simulink model "part_2_no_coulomb_friction"  (R2019a)
settings: Solver=VariableStepAuto  StartTime=0.0  StopTime=9  RelTol=1e-3
settings Model: Creator=Matthew Frantz  LastModifiedBy=Matthew Frantz
settings SolverCC: ZeroCrossAlgorithm=Adaptive
settings DebuggingCC: IgnoredZcDiagnostic=none

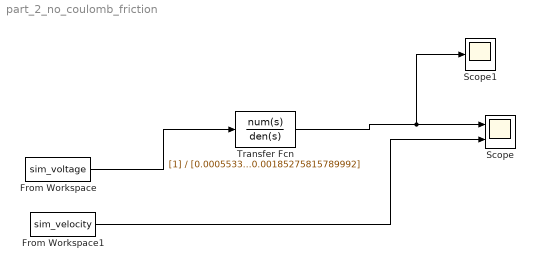
== system part_2_no_coulomb_friction ==
  From Workspace : FromWorkspace  VariableName=sim_voltage  OutDataTypeStr=double  SampleTime=0.001
  From Workspace1 : FromWorkspace  VariableName=sim_velocity  SampleTime=0.001
  Scope : Scope  NumInputPorts=2
  Scope1 : Scope
  Transfer Fcn : TransferFcn  Denominator=[0.000553342193254858 0.00185275815789992]
  wires:
  Transfer Fcn/1 -> Scope1/1, Scope/1
  From Workspace1/1 -> Scope/2
  From Workspace/1 -> Transfer Fcn/1
